simulink library "outp"  (R2021b)
settings: Solver=VariableStepAuto  StartTime=0.0  StopTime=10.0  RelTol=1e-3
undefined symbols (not defined in the file): ENUM_PMMMODE_CHARGE, ENUM_PMMMODE_IDLE, ENUM_PMMMODE_INITIALIZE, ENUM_PMMMODE_POWERDOWN, ENUM_PMMMODE_SLEEP, Left, outp, slcm, TRUE
libraries: FVT_lib x1177, hcu_lib x4, simulink x1
(part 4 of 11)

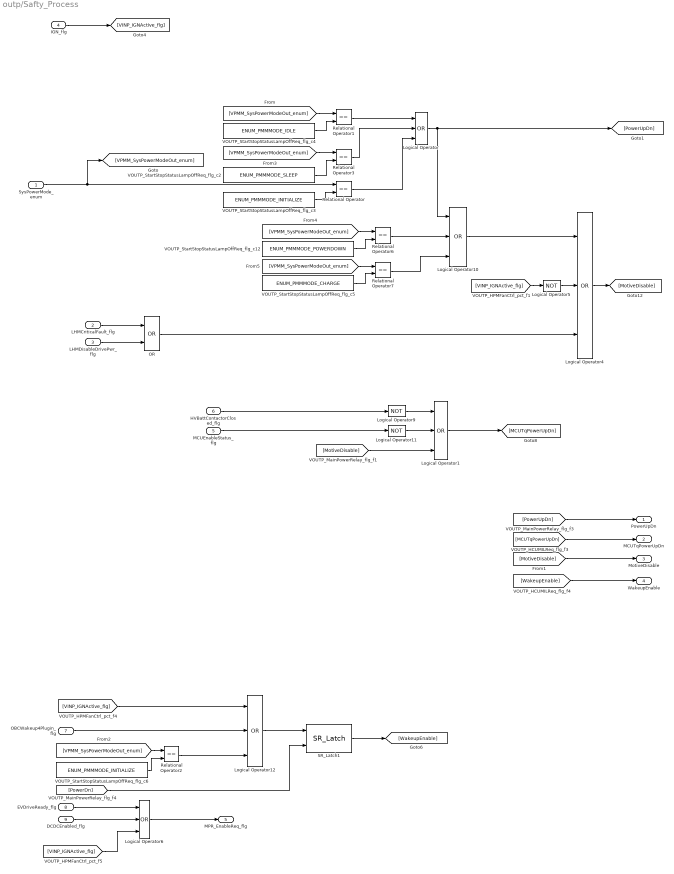
== system outp/Safty_Process ==
  SysPowerMode_enum : Inport
  LHMCriticalFault_flg : Inport  Port=2
  LHMDisableDrivePwr_flg : Inport  Port=3
  IGN_flg : Inport  Port=4
  MCUEnableStatus_flg : Inport  Port=5
  HVBattContactorClosed_flg : Inport  Port=6
  OBCWakeup4Plugin_flg : Inport  Port=7
  EVDriveReady_flg : Inport  Port=8
  DCDCEnabled_flg : Inport  Port=9
  Logical Operator{,1,4,6,10,12} (6 alike) : Logic  Operator=OR  Inputs=3  AllPortsSameDT=off  OutDataTypeStr=boolean
  Logical Operator11 : Logic  Operator=NOT  AllPortsSameDT=off  OutDataTypeStr=boolean
  Logical Operator5 : Logic  Operator=NOT  AllPortsSameDT=off  OutDataTypeStr=boolean
  Logical Operator9 : Logic  Operator=NOT  AllPortsSameDT=off  OutDataTypeStr=boolean
  OR : Logic  Operator=OR  AllPortsSameDT=off  OutDataTypeStr=boolean
  Relational Operator{,1..3,6..7} (6 alike) : RelationalOperator  Operator===  OutDataTypeStr=boolean  RndMeth=Nearest
  SR_Latch1 : hcu_lib/Basic_Blocks/SR_Latch
      settings: SourceProductName=HCU Relative Block Library
  VOUTP_StartStopStatusLampOffReq_flg_c12 : Constant  Value=ENUM_PMMMODE_POWERDOWN
  VOUTP_StartStopStatusLampOffReq_flg_c2 : Constant  Value=ENUM_PMMMODE_SLEEP
  VOUTP_StartStopStatusLampOffReq_flg_c3 : Constant  Value=ENUM_PMMMODE_INITIALIZE
  VOUTP_StartStopStatusLampOffReq_flg_c4 : Constant  Value=ENUM_PMMMODE_IDLE
  VOUTP_StartStopStatusLampOffReq_flg_c5 : Constant  Value=ENUM_PMMMODE_CHARGE
  VOUTP_StartStopStatusLampOffReq_flg_c6 : Constant  Value=ENUM_PMMMODE_INITIALIZE
  PowerUpDn : Outport
  MCUTqPowerUpDn : Outport  Port=2
  MotiveDisable : Outport  Port=3
  WakeupEnable : Outport  Port=4
  MPR_EnableReq_flg : Outport  Port=5
  wires:
  [VINP_IGNActive_flg] -> Logical Operator6/3
  Logical Operator6/1 -> MPR_EnableReq_flg/1
  DCDCEnabled_flg/1 -> Logical Operator6/2
  EVDriveReady_flg/1 -> Logical Operator6/1
  Relational Operator2/1 -> Logical Operator12/3
  [VPMM_SysPowerModeOut_enum] -> Relational Operator2/1
  VOUTP_StartStopStatusLampOffReq_flg_c6/1 -> Relational Operator2/2
  SR_Latch1/1 -> [WakeupEnable]
  [PowerDn] -> SR_Latch1/2
  Logical Operator12/1 -> SR_Latch1/1
  [VINP_IGNActive_flg] -> Logical Operator12/1
  OBCWakeup4Plugin_flg/1 -> Logical Operator12/2
  [WakeupEnable] -> WakeupEnable/1
  [MCUTqPowerUpDn] -> MCUTqPowerUpDn/1
  [PowerUpDn] -> PowerUpDn/1
  IGN_flg/1 -> [VINP_IGNActive_flg]
  HVBattContactorClosed_flg/1 -> Logical Operator9/1
  Logical Operator9/1 -> Logical Operator1/1
  [MotiveDisable] -> Logical Operator1/3
  Logical Operator1/1 -> [MCUTqPowerUpDn]
  Logical Operator11/1 -> Logical Operator1/2
  MCUEnableStatus_flg/1 -> Logical Operator11/1
  Logical Operator10/1 -> Logical Operator4/1
  Relational Operator/1 -> Logical Operator/3
  Relational Operator6/1 -> Logical Operator10/2
  [VPMM_SysPowerModeOut_enum] -> Relational Operator6/1
  VOUTP_StartStopStatusLampOffReq_flg_c12/1 -> Relational Operator6/2
  Logical Operator4/1 -> [MotiveDisable]
  Logical Operator5/1 -> Logical Operator4/2
  [VINP_IGNActive_flg] -> Logical Operator5/1
  Logical Operator/1 -> Logical Operator10/1, [PowerUpDn]
  [VPMM_SysPowerModeOut_enum] -> Relational Operator1/1
  VOUTP_StartStopStatusLampOffReq_flg_c4/1 -> Relational Operator1/2
  VOUTP_StartStopStatusLampOffReq_flg_c3/1 -> Relational Operator/2
  SysPowerMode_enum/1 -> Relational Operator/1, [VPMM_SysPowerModeOut_enum]
  LHMCriticalFault_flg/1 -> OR/1
  LHMDisableDrivePwr_flg/1 -> OR/2
  OR/1 -> Logical Operator4/3
  Relational Operator1/1 -> Logical Operator/1
  Relational Operator3/1 -> Logical Operator/2
  VOUTP_StartStopStatusLampOffReq_flg_c2/1 -> Relational Operator3/2
  [VPMM_SysPowerModeOut_enum] -> Relational Operator3/1
  VOUTP_StartStopStatusLampOffReq_flg_c5/1 -> Relational Operator7/2
  [VPMM_SysPowerModeOut_enum] -> Relational Operator7/1
  Relational Operator7/1 -> Logical Operator10/3
  [MotiveDisable] -> MotiveDisable/1

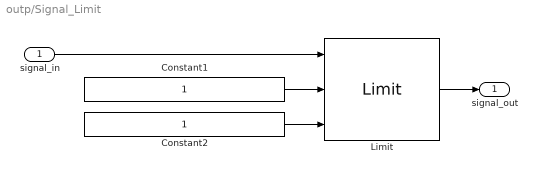
== system outp/Signal_Limit ==
  signal_in : Inport
  Constant1 : Constant
  Constant2 : Constant
  Limit : hcu_lib/Basic_Blocks/Limit
      settings: SourceProductName=HCU Relative Block Library
  signal_out : Outport
  wires:
  Constant1/1 -> Limit/2
  Constant2/1 -> Limit/3
  signal_in/1 -> Limit/1
  Limit/1 -> signal_out/1

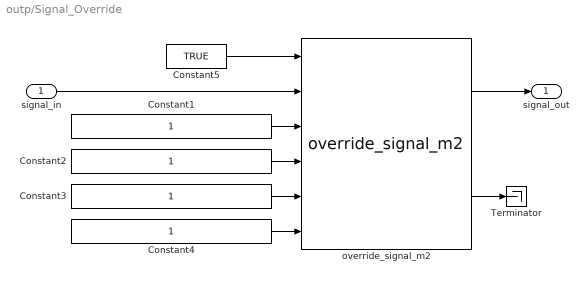
== system outp/Signal_Override ==
  signal_in : Inport
  Constant{1..4} (4 alike) : Constant
  Constant5 : Constant  Value=TRUE
  Terminator : Terminator
  "override_signal_m2 " : hcu_lib/Signal_Process_Blocks/override_signal_m2 
      settings: SourceProductName=HCU Relative Block Library
  signal_out : Outport
  wires:
  Constant1/1 -> "override_signal_m2 "/3
  Constant2/1 -> "override_signal_m2 "/4
  Constant3/1 -> "override_signal_m2 "/5
  Constant4/1 -> "override_signal_m2 "/6
  Constant5/1 -> "override_signal_m2 "/1
  "override_signal_m2 "/2 -> Terminator/1
  signal_in/1 -> "override_signal_m2 "/2
  "override_signal_m2 "/1 -> signal_out/1

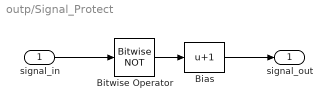
== system outp/Signal_Protect ==
  signal_in : Inport
  Bias : Bias  Bias=1
  Bitwise Operator : simulink/Logic and Bit Operations/Bitwise Operator  logicop=NOT  UseBitMask=off  BitMask=bin2dec('11011001')  BitMaskRealWorld=Stored Integer
  signal_out : Outport
  wires:
  Bitwise Operator/1 -> Bias/1
  Bias/1 -> signal_out/1
  signal_in/1 -> Bitwise Operator/1

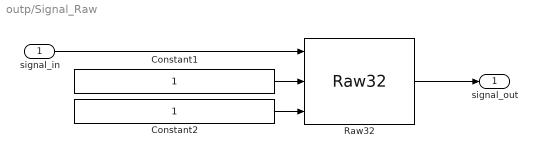
== system outp/Signal_Raw ==
  signal_in : Inport
  Constant1 : Constant
  Constant2 : Constant
  Raw32 : hcu_lib/Signal_Conversion_Blocks/Raw32
      settings: SourceProductName=HCU Relative Block Library
  signal_out : Outport
  wires:
  Constant1/1 -> Raw32/2
  Constant2/1 -> Raw32/3
  signal_in/1 -> Raw32/1
  Raw32/1 -> signal_out/1

== system outp/Model Info/EmptySubsystem ==
